simulink model "ControlRetroEstadosEscalon"  (R2017b)
settings: Solver=ode45  StartTime=0.0  StopTime=100  RelTol=1e-3
values from neighbouring files (symbols this model uses):
  A = double(A)    [Linealizacion.m]
  B = double(B)    [Linealizacion.m]
  C = double(C)    [Linealizacion.m]
  K = acker(Agorrito,Bgorrito,roots(PD))    [Linealizacion.m]
  K1 = acker(Agorrito1,Bgorrito1,roots(PD1))    [Linealizacion.m]
  K2 = acker(Agorrito2,Bgorrito2,roots(PD2))    [Linealizacion.m]
  L1 = acker(A',C',roots(PDobs))'    [Linealizacion.m]
settings Model: Creator=Cx001la  LastModifiedBy=Cx001la

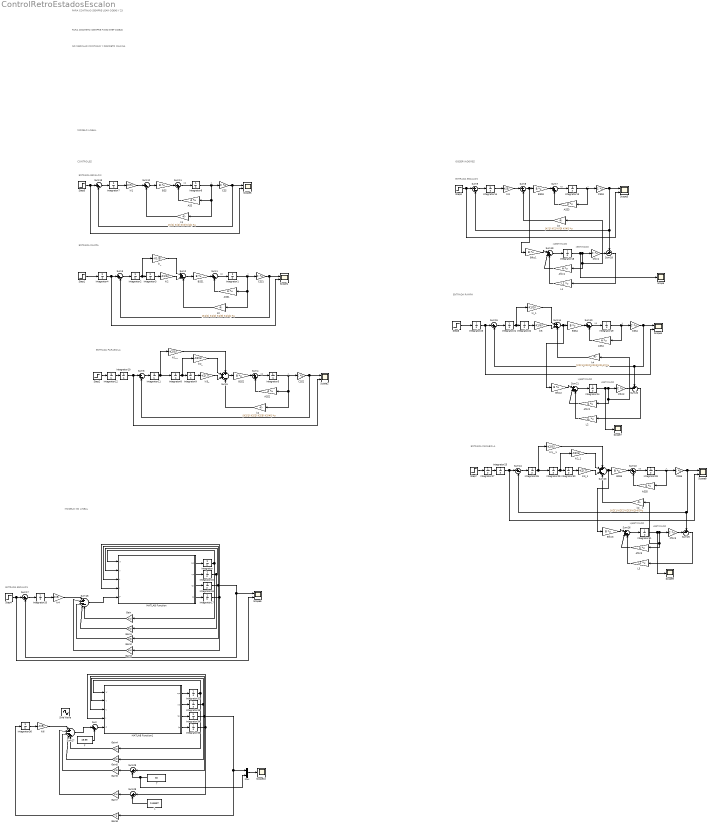
== system ControlRetroEstadosEscalon ==
  note: MODELO LINEAL
  note: PARA DISCRETO SIEMPRE FIXED STEP ODE45
  note: OBSERVADORES
  note: ENTRADA ESCALON
  note: xp
  note: x
  note: ENTRADA RAMPA
  note: x
  note: xp
  note: x
  note: ENTRADA PARABOLA
  note: xp
  note: CONTROLES
  note: ENTRADA ESCALON
  note: x
  note: xp
  note: xpESTIMADO
  note: xESTIMADO
  note: PARA CONTINUO SIEMPRE USAR ODE45 Y 23
  note: NO MEZCLAR CONTINUO Y DISCRETO MAKINA
  note: MODELO NO LINEAL
  note: ENTRADA ESCALON
  note: x
  note: xp
  note: ENTRADA RAMPA
  note: xESTIMADO
  note: xpESTIMADO
  note: x
  note: xp
  note: ENTRADA PARABOLA
  note: xpESTIMADO
  note: xESTIMADO
  ASS{,1..5} (6 alike) : Gain  Gain=A  Multiplication=Matrix(K*u)
  Afcc1 : Gain  Gain=A  Multiplication=Matrix(K*u)
  Afcc2 : Gain  Gain=A  Multiplication=Matrix(K*u)
  Afcc3 : Gain  Gain=A  Multiplication=Matrix(K*u)
  BSS{,1..5} (6 alike) : Gain  Gain=B  Multiplication=Matrix(K*u)
  Bfcc1 : Gain  Gain=B  Multiplication=Matrix(K*u)
  Bfcc2 : Gain  Gain=B  Multiplication=Matrix(K*u)
  Bfcc3 : Gain  Gain=B  Multiplication=Matrix(K*u)
  CSS{,1..5} (6 alike) : Gain  Gain=C  Multiplication=Matrix(K*u)
  Cfcc1 : Gain  Gain=C  Multiplication=Matrix(K*u)
  Cfcc2 : Gain  Gain=C  Multiplication=Matrix(K*u)
  Cfcc3 : Gain  Gain=C  Multiplication=Matrix(K*u)
  F : Constant  Value=19.99
  Gain : Gain  Gain=K(1)
  Gain1 : Gain  Gain=K(2)
  Gain2 : Gain  Gain=K(3)
  Gain3 : Gain  Gain=K(4)
  Gain4 : Gain  Gain=K(1)
  Gain5 : Gain  Gain=K(2)
  Gain6 : Gain  Gain=K(3)
  Gain7 : Gain  Gain=K(4)
  Gain8 : Gain  Gain=-1
  Integrator : Integrator  InitialCondition=0.1
  Integrator{1..16,18..31,33..34,36} (33 alike) : Integrator
  Integrator17 : Integrator  InitialCondition=0.001
  Integrator32 : Integrator  InitialCondition=0.01
  Integrator35 : Integrator  InitialCondition=0.000000001
  L : Constant  Value=0.48487
  L1 : Gain  Gain=L1  Multiplication=Matrix(K*u)
  L2 : Gain  Gain=L1  Multiplication=Matrix(K*u)
  L3 : Gain  Gain=L1  Multiplication=Matrix(K*u)
  MATLAB Function : MATLAB Function  TreatAsAtomicUnit=on
  MATLAB Function1 : MATLAB Function  TreatAsAtomicUnit=on
  Mux : Mux  Inputs=2
  Scope{,7,9..10} (4 alike) : Scope
  Scope{1..6,8} (7 alike) : Scope  NumInputPorts=2
  Sine Wave : Sin  SampleTime=0
  Step{1..7} (7 alike) : Step  Time=0  SampleTime=0
  Sum{,1,4,7,10..11,22} (7 alike) : Sum  Inputs=|++
  Sum{3,6,8..9,12..13,15,17,24,28..29} (11 alike) : Sum  Inputs=|+-
  Sum14 : Sum  Inputs=|++-
  Sum16 : Sum  Inputs=|+----
  Sum18 : Sum  Inputs=+-|
  Sum19 : Sum  Inputs=|+++
  Sum2 : Sum  Inputs=|++-
  Sum20 : Sum  Inputs=+-|
  Sum21 : Sum  Inputs=|+++
  Sum23 : Sum  Inputs=+++-
  Sum25 : Sum  Inputs=+-|
  Sum26 : Sum  Inputs=|+++
  Sum27 : Sum  Inputs=|+----
  Sum5 : Sum  Inputs=+++-
  T : Constant  Value=30
  k1 : Gain  Gain=[K(1) K(2) K(3) K(4)]  Multiplication=Matrix(K*u)
  k2 : Gain  Gain=[K1(1) K1(2) K1(3) K1(4)]  Multiplication=Matrix(K*u)
  k2__ : Gain  Gain=[K2(1) K2(2) K2(3) K2(4)]  Multiplication=Matrix(K*u)
  k2__1 : Gain  Gain=[K2(1) K2(2) K2(3) K2(4)]  Multiplication=Matrix(K*u)
  k3 : Gain  Gain=[K(1) K(2) K(3) K(4)]  Multiplication=Matrix(K*u)
  k4 : Gain  Gain=[K1(1) K1(2) K1(3) K1(4)]  Multiplication=Matrix(K*u)
  ki{1,3..4,6} (4 alike) : Gain  Gain=-K(5)
  ki1__ : Gain  Gain=-K2(5)
  ki1__1 : Gain  Gain=-K2(5)
  ki2 : Gain  Gain=-K1(6)
  ki2_ : Gain  Gain=-K2(6)
  ki2_1 : Gain  Gain=-K2(6)
  ki3_ : Gain  Gain=-K2(7)
  ki3_1 : Gain  Gain=-K2(7)
  ki5 : Gain  Gain=-K1(6)
  ki_ : Gain  Gain=-K1(5)
  ki_1 : Gain  Gain=-K1(5)
  wires:
  ASS/1 -> Sum11/2
  Sum13/1 -> Integrator7/1
  ki1/1 -> Sum12/1
  Sum12/1 -> BSS/1
  k1/1 -> Sum12/2
  Integrator7/1 -> ki1/1
  BSS/1 -> Sum11/1
  Step5/1 -> Scope5/2, Sum13/1
  Integrator6/1 -> k1/1, ASS/1, CSS/1
  Sum11/1 -> Integrator6/1
  CSS/1 -> Scope5/1, Sum13/2
  Sum1/1 -> Integrator1/1
  CSS1/1 -> Scope1/1, Sum3/2
  BSS1/1 -> Sum1/1
  Sum2/1 -> BSS1/1
  Sum3/1 -> Integrator2/1
  ASS1/1 -> Sum1/2
  Integrator1/1 -> k2/1, ASS1/1, CSS1/1
  Integrator3/1 -> ki2/1
  Integrator2/1 -> ki_/1, Integrator3/1
  k2/1 -> Sum2/3
  ki2/1 -> Sum2/2
  ki_/1 -> Sum2/1
  Integrator4/1 -> Scope1/2, Sum3/1
  Step1/1 -> Integrator4/1
  Integrator9/1 -> ki3_/1
  ASS2/1 -> Sum4/2
  Integrator5/1 -> k2__/1, ASS2/1, CSS2/1
  Sum6/1 -> Integrator11/1
  Sum5/1 -> BSS2/1
  BSS2/1 -> Sum4/1
  CSS2/1 -> Scope2/1, Sum6/2
  Sum4/1 -> Integrator5/1
  Step2/1 -> Integrator12/1
  Integrator10/1 -> Scope2/2, Sum6/1
  Integrator8/1 -> ki2_/1, Integrator9/1
  Integrator11/1 -> ki1__/1, Integrator8/1
  ki1__/1 -> Sum5/1
  k2__/1 -> Sum5/4
  ki3_/1 -> Sum5/3
  ki2_/1 -> Sum5/2
  Integrator12/1 -> Integrator10/1
  Sum7/1 -> Integrator13/1
  Step3/1 -> Scope3/2, Sum9/1
  BSS3/1 -> Sum7/1
  ki3/1 -> Sum8/1
  k3/1 -> Sum8/2
  Integrator14/1 -> ki3/1
  Sum9/1 -> Integrator14/1
  ASS3/1 -> Sum7/2
  Integrator13/1 -> ASS3/1, CSS3/1
  Sum19/1 -> Integrator18/1
  Sum8/1 -> Bfcc1/1, BSS3/1
  CSS3/1 -> Scope3/1, Sum18/1, Sum9/2
  Sum18/1 -> L1/1
  Integrator18/1 -> Scope/1, k3/1, Afcc1/1, Cfcc1/1
  Cfcc1/1 -> Sum18/2
  Afcc1/1 -> Sum19/2
  L1/1 -> Sum19/3
  Bfcc1/1 -> Sum19/1
  MATLAB Function/1(wp) -> Integrator/1
  MATLAB Function/2(vp) -> Integrator15/1
  MATLAB Function/3(tp) -> Integrator16/1
  MATLAB Function/4(lp) -> Integrator17/1
  Integrator/1 -> MATLAB Function/1(w), Gain/1
  Integrator15/1 -> Gain1/1, MATLAB Function/2(v)
  Integrator16/1 -> Sum17/2, Scope6/1, Gain2/1, MATLAB Function/3(t)
  Integrator17/1 -> Gain3/1, MATLAB Function/4(l)
  Sum17/1 -> Integrator20/1
  Step4/1 -> Scope6/2, Sum17/1
  Sum16/1 -> MATLAB Function/5(F)
  Integrator20/1 -> ki4/1
  ki4/1 -> Sum16/1
  Gain/1 -> Sum16/5
  Gain1/1 -> Sum16/4
  Gain2/1 -> Sum16/3
  Gain3/1 -> Sum16/2
  ki_1/1 -> Sum14/1
  Integrator21/1 -> ki_1/1, Integrator22/1
  Integrator23/1 -> Scope4/2, Sum15/1
  k4/1 -> Sum14/3
  Integrator19/1 -> ASS4/1, CSS4/1
  Step6/1 -> Integrator23/1
  ki5/1 -> Sum14/2
  BSS4/1 -> Sum10/1
  ASS4/1 -> Sum10/2
  Sum15/1 -> Integrator21/1
  Sum10/1 -> Integrator19/1
  Integrator22/1 -> ki5/1
  CSS4/1 -> Scope4/1, Sum20/1, Sum15/2
  Bfcc2/1 -> Sum21/1
  Sum14/1 -> Bfcc2/1, BSS4/1
  Cfcc2/1 -> Sum20/2
  Integrator24/1 -> Scope7/1, k4/1, Afcc2/1, Cfcc2/1
  L2/1 -> Sum21/3
  Afcc2/1 -> Sum21/2
  Sum21/1 -> Integrator24/1
  Sum20/1 -> L2/1
  k2__1/1 -> Sum23/4
  Integrator30/1 -> ki3_1/1
  Integrator29/1 -> ki2_1/1, Integrator30/1
  Integrator26/1 -> ki1__1/1, Integrator29/1
  ki3_1/1 -> Sum23/3
  Step7/1 -> Integrator27/1
  Integrator25/1 -> Scope8/2, Sum24/1
  ki1__1/1 -> Sum23/1
  Integrator28/1 -> ASS5/1, CSS5/1
  Sum24/1 -> Integrator26/1
  ki2_1/1 -> Sum23/2
  Sum22/1 -> Integrator28/1
  ASS5/1 -> Sum22/2
  BSS5/1 -> Sum22/1
  Integrator27/1 -> Integrator25/1
  CSS5/1 -> Scope8/1, Sum24/2, Sum25/1
  Sum26/1 -> Integrator31/1
  L3/1 -> Sum26/3
  Integrator31/1 -> Scope9/1, k2__1/1, Afcc3/1, Cfcc3/1
  Cfcc3/1 -> Sum25/2
  Sum25/1 -> L3/1
  Afcc3/1 -> Sum26/2
  Bfcc3/1 -> Sum26/1
  Sum23/1 -> Bfcc3/1, BSS5/1
  ki6/1 -> Sum27/1
  Gain7/1 -> Sum27/2
  Gain4/1 -> Sum27/5
  Gain6/1 -> Sum27/3
  Gain5/1 -> Sum27/4
  Integrator32/1 -> Gain4/1, MATLAB Function1/1(w)
  MATLAB Function1/3(tp) -> Integrator34/1
  Integrator34/1 -> Sum29/1, Mux/1, Gain8/1, MATLAB Function1/3(t)
  MATLAB Function1/1(wp) -> Integrator32/1
  Integrator36/1 -> ki6/1
  Integrator33/1 -> Gain5/1, MATLAB Function1/2(v)
  MATLAB Function1/4(lp) -> Integrator35/1
  MATLAB Function1/2(vp) -> Integrator33/1
  Gain8/1 -> Integrator36/1
  Sum/1 -> MATLAB Function1/5(F)
  Sum27/1 -> Sum/1
  F/1 -> Sum/2
  Sum29/1 -> Gain6/1
  Sum28/1 -> Gain7/1
  Integrator35/1 -> Sum28/1, MATLAB Function1/4(l)
  T/1 -> Mux/2, Sum29/2
  L/1 -> Sum28/2
  Mux/1 -> Scope10/1

== matlab function ControlRetroEstadosEscalon/MATLAB Function1 ==
  data: w input; wp output; v input; t input; l input; F input; vp output; tp output; lp output
function [wp,vp,tp,lp] = fcn(w,v,t,l,F)
time=0; a=0; wn=0; 
g=9.81; lo=0.5; k=100; m=1;
wp=(1/l)*(  -2*v*w -(a*wn^2*sin(wn*time)-g)*sin(t)  +F*l );
vp=l*w   -(k/m)*(l-lo)   -(  g-a*wn^2*sin(wn*time)  )*cos(t);
tp=w;
lp=v;

== matlab function ControlRetroEstadosEscalon/MATLAB Function ==
  data: w input; wp output; v input; t input; l input; F input; vp output; tp output; lp output
function [wp,vp,tp,lp] = fcn(w,v,t,l,F)
time=0; a=0; wn=0; 
g=9.81; lo=0.5; k=100; m=1;
wp=(1/l)*(  -2*v*w -(a*wn^2*sin(wn*time)-g)*sin(t)  +F*l );
vp=l*w   -(k/m)*(l-lo)   -(  g-a*wn^2*sin(wn*time)  )*cos(t);
tp=w;
lp=v;
